simulink model "Ass_1"  (R2024b)
settings: Solver=FixedStepAuto  StartTime=time_cmd(1)  StopTime=time_cmd(end)  FixedStep=1/f_cmd  RelTol=1e-3
model workspace (MAT data in the model file):
  SL_ROS_VariableLengthArrays_MaxSizes.CommonInfo.ArrayTruncateAction = 'EmitWarning'
  SL_ROS_VariableLengthArrays_MaxSizes.MsgTypeMap = containers.Map
  SL_ROS_VariableLengthArrays_MaxSizes.MsgTypeMap.serialization.keys = {'sensor_msgs/LaserScan'}
  SL_ROS_VariableLengthArrays_MaxSizes.MsgTypeMap.serialization.values{1}(1).PropertyName = 'Intensities'
  SL_ROS_VariableLengthArrays_MaxSizes.MsgTypeMap.serialization.values{1}(1).DataType = 'single'
  SL_ROS_VariableLengthArrays_MaxSizes.MsgTypeMap.serialization.values{1}(1).MaxLength = 360
  SL_ROS_VariableLengthArrays_MaxSizes.MsgTypeMap.serialization.values{1}(2).PropertyName = 'Ranges'
  SL_ROS_VariableLengthArrays_MaxSizes.MsgTypeMap.serialization.values{1}(2).DataType = 'single'
  SL_ROS_VariableLengthArrays_MaxSizes.MsgTypeMap.serialization.values{1}(2).MaxLength = 360
  SL_ROS_VariableLengthArrays_MaxSizes.MsgTypeMap.serialization.uniformity = 0
  SL_ROS_VariableLengthArrays_MaxSizes.MsgTypeMap.serialization.keyType = 'char'
  SL_ROS_VariableLengthArrays_MaxSizes.MsgTypeMap.serialization.valueType = 'any'
values from neighbouring files (symbols this model uses):
  f_cmd = round(f_odom)    [Main_Ass_1.m]
undefined symbols (not defined in the file or in its folder): Angular, Linear
libraries: robotlib x5
settings Model: Creator=vise  LastModifiedBy=vise
settings OptimizationCC: DefaultParameterBehavior=Inlined  EnhancedBackFolding=on  PassReuseOutputArgsAs=Individual arguments  ZeroExternalMemoryAtStartup=off  ZeroInternalMemoryAtStartup=off  MaxStackSize=64  OptimizeBlockOrder=speed  DifferentSizesBufferReuse=on  OptimizationCustomize=off  EfficientTunableParamExpr=on
settings DebuggingCC: ParameterTunabilityLossMsg=error
settings HardwareCC: ProdBitPerPointer=32  ProdBitPerSizeT=32  ProdBitPerPtrDiffT=32  ProdLargestAtomicFloat=None  ProdIntDivRoundTo=Undefined  ProdEndianess=Unspecified  ProdWordSize=32  ProdHWDeviceType=Generic->Unspecified (assume 32-bit Generic)  UseEmbeddedCoderFeatures=off
settings SFSimCC: MATLABDynamicMemAlloc=off
settings RTWCC: Description=Embedded Coder  SystemTargetFile=ert.tlc  HardwareBoard=Robot Operating System (ROS)  TLCOptions="-aInlineSetEventsForThisBaseRateFcn=TLC_FALSE -aSuppressMultiTaskScheduler=TLC_FALSE  -aRateBasedStepFcn=0"  TemplateMakefile=ert_default_tmf  Toolchain=Catkin  TargetLang=C++
settings CodeAppCC: ForceParamTrailComments=on  IgnoreCustomStorageClasses=off  OperatorAnnotations=on  SimulinkDataObjDesc=on  SFDataObjDesc=on  InsertBlockDesc=on
settings ERTTargetCC: SupportNonInlinedSFcns=on

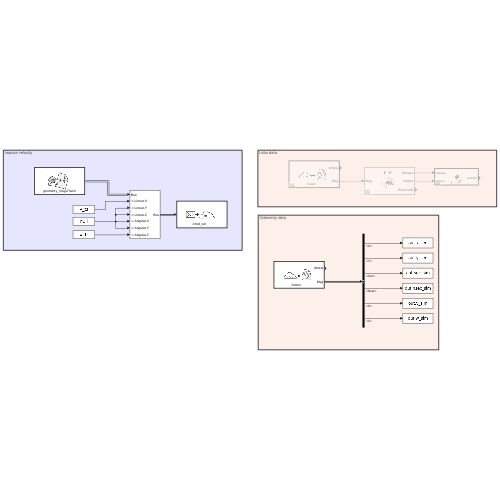
[thumbnail: Simulink's stored preview of the top-level diagram]
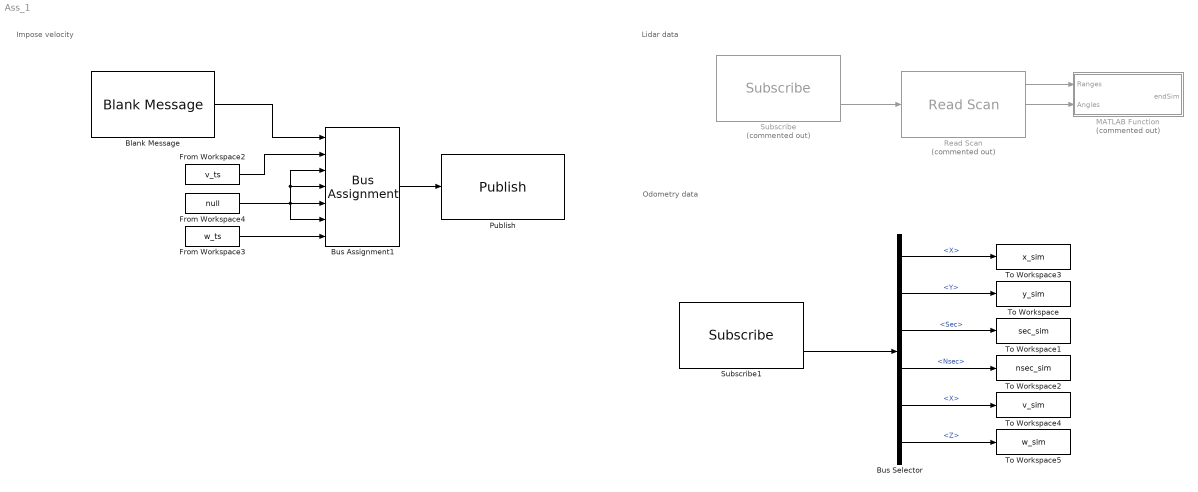
== system Ass_1 ==
  note: Odometry data
  note: Lidar data
  note: Impose velocity
  Blank Message : robotlib/Blank Message  messageClass=Message  entityType=geometry_msgs/Twist  messageType=geometry_msgs/Twist  SampleTime=1/f_cmd  legacyBusStruct=off
  Bus Assignment1 : BusAssignment  AssignedSignals=Linear.X,Linear.Y,Linear.Z,Angular.X,Angular.Y,Angular.Z
  Bus Selector : BusSelector  OutputSignals=Pose.Pose.Position.X,Pose.Pose.Position.Y,Header.Stamp.Sec,Header.Stamp.Nsec,Twist.Twist.Linear.X,Twist.Twist.Angular.Z
  From Workspace2 : FromWorkspace  VariableName=v_ts  SampleTime=1/f_cmd
  From Workspace3 : FromWorkspace  VariableName=w_ts  SampleTime=1/f_cmd
  From Workspace4 : FromWorkspace  VariableName=null  SampleTime=1/f_cmd
  MATLAB Function : MATLAB Function  Commented=on  TreatAsAtomicUnit=on
  Publish : robotlib/Publish  topicSource=Select from ROS network  topic=/cmd_vel  messageType=geometry_msgs/Twist  legacyBusStruct=off  messageQueueLength=1
  Read Scan : robotlib/Read Scan  Commented=on  MaximumArrayLength=360  ShowAnglesOutput=on  ShowIntensityOutput=off  ShowErrorCodeOutput=on  VariableSizeOutputs=off
  Subscribe : robotlib/Subscribe  Commented=on  topicSource=Select from ROS network  topic=/scan  messageType=sensor_msgs/LaserScan  SampleTime=-1  legacyBusStruct=off  messageQueueLength=1
  Subscribe1 : robotlib/Subscribe  topicSource=Select from ROS network  topic=/odom  messageType=nav_msgs/Odometry  SampleTime=1/f_cmd  legacyBusStruct=off  messageQueueLength=1
  To Workspace : ToWorkspace  VariableName=y_sim  SampleTime=-1
      settings: Save2DSignal=2-D array (concatenate along first dimension)
  To Workspace1 : ToWorkspace  VariableName=sec_sim  SampleTime=-1
      settings: Save2DSignal=2-D array (concatenate along first dimension)
  To Workspace2 : ToWorkspace  VariableName=nsec_sim  SampleTime=-1
      settings: Save2DSignal=2-D array (concatenate along first dimension)
  To Workspace3 : ToWorkspace  VariableName=x_sim  SampleTime=-1
      settings: Save2DSignal=2-D array (concatenate along first dimension)
  To Workspace4 : ToWorkspace  VariableName=v_sim  SampleTime=-1
      settings: Save2DSignal=2-D array (concatenate along first dimension)
  To Workspace5 : ToWorkspace  VariableName=w_sim  SampleTime=-1
      settings: Save2DSignal=2-D array (concatenate along first dimension)
  wires:
  Bus Assignment1/1 -> Publish/1
  Blank Message/1 -> Bus Assignment1/1
  From Workspace4/1 -> Bus Assignment1/6, Bus Assignment1/5, Bus Assignment1/4, Bus Assignment1/3
  Subscribe/2 -> Read Scan/1
  Read Scan/1 -> MATLAB Function/1(Ranges)
  Read Scan/2 -> MATLAB Function/2(Angles)
  From Workspace2/1 -> Bus Assignment1/2
  From Workspace3/1 -> Bus Assignment1/7
  Bus Selector/1 -> To Workspace3/1  "<X>"
  Bus Selector/2 -> To Workspace/1  "<Y>"
  Bus Selector/3 -> To Workspace1/1  "<Sec>"
  Bus Selector/4 -> To Workspace2/1  "<Nsec>"
  Bus Selector/6 -> To Workspace5/1  "<Z>"
  Bus Selector/5 -> To Workspace4/1  "<X>"
  Subscribe1/2 -> Bus Selector/1

== matlab function Ass_1/MATLAB Function ==
  data: Ranges input; endSim output; Angles input
function endSim = plotXY(Ranges,Angles)

% Takes as input "Read Scan" block output and processes it to create a plot in
% global XY reference. Only starts when at least some data different from 
% zero are provided (i.e. when the subscriber outputs a message).

endSim = any(Ranges>0);

if endSim

    x = Ranges.*cos(Angles);
    y = Ranges.*sin(Angles);

    xValid = x(isfinite(x));
    yValid = y(isfinite(y));
    
    plot(xValid,yValid,'.','MarkerSize',8)
    title('Laser scan')
    grid on
    xlabel('X')
    ylabel('Y')
    set(gca,'Ydir','reverse')   % invert Y axis
    axis equal
    xlim([-5 5])
    ylim([-5 5])
    view([90 -90])

end
